simulink model "funkcia1"  (R2020a)
settings: Solver=VariableStepAuto  StartTime=0.0  StopTime=10.0  RelTol=1e-3
libraries: simulink x1
settings Model: Creator=xacha  LastModifiedBy=xacha

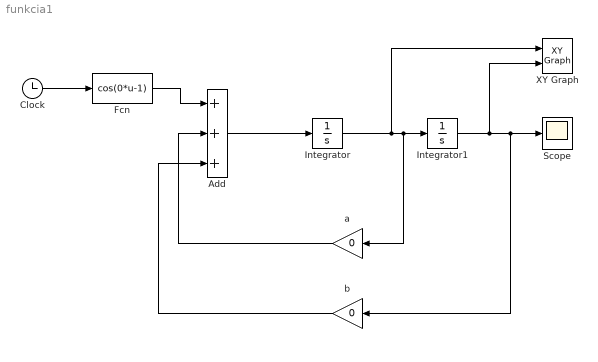
== system funkcia1 ==
  Add : Sum  Inputs=+++
  Clock : Clock
  Fcn : Fcn  Expr=cos(0*u-1)
  Integrator : Integrator
  Integrator1 : Integrator
  Scope : Scope
  XY Graph : simulink/Sinks/XY Graph  xmin=-1  xmax=1  ymin=-1  ymax=1  st=-1
  a : Gain  Gain=0
  b : Gain  Gain=0
  wires:
  Clock/1 -> Fcn/1
  Fcn/1 -> Add/1
  Add/1 -> Integrator/1
  Integrator/1 -> XY Graph/1, a/1, Integrator1/1
  Integrator1/1 -> XY Graph/2, b/1, Scope/1
  a/1 -> Add/2
  b/1 -> Add/3
